simulink library "carnotUIBK"  (R2018b)
settings: Solver=VariableStepAuto  StartTime=0.0  StopTime=10.0  RelTol=1e-3  EnableMultiTasking=on
values from neighbouring files (symbols this model uses):
  A = 7*10*2    (= 140)    [theta_ground_v1.m]    (also in xlswrite1.m = num2cell(data))
  amb_factor = 1    [DOOR.m]    (also in WALL.m; WINDOW.m = 0)
  area = obj.width * obj.height    [DOOR.m]    (also in RES.m = []; ROOM.m = 0; THERMALZONE.m = area + room(kk).area; WALL.m = area - obj.doors(jj).calc_area())
  B = A/(0.5 * P)    (= 8.23529411765)    [theta_ground_v1.m]
  boundary = BOUNDARY()    [BUILDING.m]    (also in WALL.m = '')
  building = obj    [BUILDING.m]    (also in create_building_automatic.m = building.save(); ini_building_automatic.m = building.add_variant_hvac(building.variant_hvac, hvac); load_building_automatic.m = building.save())
  C = zeros(1,length(d)+1)    [CONSTRUCTION.m]    (also in DOOR.m = [0 0 0]; WALL.m = [0 0 0]; WINDOW.m = [0 0 0])
  control = 2    [GAIN.m]    (also in GAINS.m)
  cp = str2num(value)    [CONSTRUCTION.m]
  height = 0    [DOOR.m]    (also in ROOM.m; THERMALZONE.m; WALL.m; WINDOW.m)
  p = [timevec_weather weather(:,12)]    [BOUNDARY.m]    (also in WEATHER.m = 0; init_carnotUIBK.m = cell2mat(carnotUIBKpaths(i,2)))
  rho = str2num(value)    [CONSTRUCTION.m]    (also in theta_ground_v1.m = 2000)
  type = 1    [CONSTRUCTION.m]    (also in GAINS.m = raw_moisture{ii,3}; STRUCTURE.m = 0)
  view_factor = 1    [DOOR.m]    (also in WINDOW.m = 0)
  wall = []    [ROOM.m]
  z = obj.Z    [WALL.m]    (also in theta_ground_v1.m = 0)
  zone = obj.zone(ind)    [THERMALZONE.m]
undefined symbols (not defined in the file or in its folder): const, Dd, get_building, pos, Qdot_C, Qdot_H, Qdot_I_electricity, Qdot_I_light, Qdot_I_person, Qdot_S, Qdot_T_ground, Qdot_T_neighbour, Qdot_T_opaque, Qdot_T_window, Qdot_V_infiltration, Qdot_V_mech, Qdot_V_window, r_frame, solar_ratio, solar_ratio1, solar_ratio2, Tc, Tr, Ts, Uvalue, wallsurface, window, window_height, window_heigth, window_width, windowsurface, x_CO2, x_H2O, x_VOC
libraries: carnot x104, simulink x16, $bdroot x16, simulink_extras x14
(part 5 of 12)

== system carnotUIBK/HVAC/HVAC_1001_electrical heaters/electrical heater zone 6 ==
  temperature setpoint : Inport
  temperature room : Inport  Port=2
  Enable : EnablePort
  " " : Constant  Value=0
  "   " : Constant  Value=zeros(1,15)
  Bus Creator1 : BusCreator  Inputs=2
  Bus Selector5 : BusSelector  OutputSignals=Ts
  Integrator : Integrator
  Mux1 : Mux  Inputs=[1 1 15 1 1]
  PID : simulink/Continuous/PID Controller  Controller=PI  Form=Ideal  TimeDomain=Continuous-time  SampleTime=-1  IntegratorMethod=Forward Euler  FilterMethod=Forward Euler  ControllerParametersSource=internal  P=Kp  I=1/(Tn*60)  D=0  UseFilter=on  N=100  TunerSelectOption=Transfer Function Based (PID Tuner App)  InitialConditionSource=internal  InitialConditionForIntegrator=0  InitialConditionForFilter=0  DifferentiatorICPrevScaledInput=0  ExternalReset=none  TrackingMode=off  Kt=1  LimitOutput=on  UpperSaturationLimit=1  LowerSaturationLimit=0  LinearizeAsGain=off  AntiWindupMode=clamping  Kb=1  POutMin=[]  POutMax=[]  IOutMin=[]  IOutMax=[]  DOutMin=[]  DOutMax=[]  NOutMin=[]  NOutMax=[]  SumOutMin=[]  SumOutMax=[]  SaturationOutMin=[]  SaturationOutMax=[]  PParamMin=[]  PParamMax=[]  IParamMin=[]  IParamMax=[]  DParamMin=[]  DParamMax=[]  NParamMin=[]  NParamMax=[]  KbParamMin=[]  KbParamMax=[]  KtParamMin=[]  KtParamMax=[]  KbOutMin=[]  KbOutMax=[]  KtOutMin=[]  KtOutMax=[]  IntegratorOutMin=[]  IntegratorOutMax=[]  FilterOutMin=[]  FilterOutMax=[]  SumI1OutMin=[]  SumI1OutMax=[]  SumI2OutMin=[]  SumI2OutMax=[]  SumI3OutMin=[]  SumI3OutMax=[]  SumI4OutMin=[]  SumI4OutMax=[]  SumDOutMin=[]  SumDOutMax=[]  DifferentiatorOutMin=[]  DifferentiatorOutMax=[]  FilterDiffOutCoefMin=[]  FilterDiffOutCoefMax=[]  ReciprocalOutMin=[]  ReciprocalOutMax=[]  SumDenOutMin=[]  SumDenOutMax=[]  SumNumOutMin=[]  SumNumOutMax=[]  DivideOutMin=[]  DivideOutMax=[]  IntegratorContinuousStateAttributes=''  IntegratorStateMustResolveToSignalObject=off  IntegratorRTWStateStorageClass=Auto  FilterContinuousStateAttributes=''  FilterStateMustResolveToSignalObject=off  FilterRTWStateStorageClass=Auto  ParallelPVariant=Passthrough  IdealPVariant=InternalParameters  IVariant=InternalParameters  DVariant=Disabled  IntegratorVariant=Continuous  SatVariant=Enabled  AWVariant=ContClampingIdeal  PCopyVariant=InternalParamsIdeal  TRVariant=Disabled  FdbkBlocksVariant=Forward  IdealPFdbkVariant=Disabled  SatFdbkVariant=Disabled  DerivativeFilterVariant=Disabled  NVariant=Disabled  NCopyVariant=Disabled_SignalSpec  FilterICVariant=Disabled  IntegratorICVariant=InternalICs  ExternalResetVariant=Disabled  TRSumVariant=Passthrough  SumFdbkVariant=Disabled  SumVariant=Sum_PI
  Product : Product
  Sum13 : Sum  Inputs=|+-
  Transfer Fcn (with initial states) : Subsystem  mask(Transfer Function with Initial States){N=[1], D=[timeconst 1], X0=0}
      mask prompts: N "Numerator:"; D "Denominator:"; X0 "Initial conditions:"
      mask help: Vector expressions for numerator, and denominator. Coefficients are in descending powers of s.
      mask init:
      | [A,B,C,Dd]=tf2ss(N,D);if (isempty(X0));[m,n]=size(A);X0=zeros(1,m); end;
      mask Help: Specify the initial states for the transfer function.  The state ordering is determined by the m-file tf2ss.  There is no unique mapping of the states in a transfer function to states in a state-space representation.  However, tf2ss will consistently use the same mapping for a given transfer function.
      mask Display: dpoly(N,D,'s')
  convective : Gain  Gain=s_conv  SaturateOnIntegerOverflow=on  OutDataTypeStr=Inherit: Same as input  ParamDataTypeStr=Inherit: Same as input
  maximal power : Constant  Value=max_power
  radiative : Gain  Gain=1-s_conv  SaturateOnIntegerOverflow=on  OutDataTypeStr=Inherit: Same as input  ParamDataTypeStr=Inherit: Same as input
  "[S]" : Outport
  "[HVAC]" : Outport  Port=2
  wires:
  Bus Creator1/1 -> "[HVAC]"/1
  Integrator/1 -> Bus Creator1/2  "heating energy"
  temperature setpoint/1 -> Sum13/1
  Bus Selector5/1 -> Sum13/2  "<Ts>"
  Product/1 -> Mux1/4, Integrator/1, Bus Creator1/1, radiative/1, convective/1  "heating power"
  "   "/1 -> Mux1/3
  radiative/1 -> Mux1/2
  temperature room/1 -> Bus Selector5/1
  maximal power/1 -> Product/2
  PID/1 -> Transfer Fcn (with initial states)/1(In1)
  convective/1 -> Mux1/1
  Mux1/1 -> "[S]"/1
  " "/1 -> Mux1/5
  Transfer Fcn (with initial states)/1(Out1) -> Product/1
  Sum13/1 -> PID/1

== system carnotUIBK/HVAC/HVAC_1001_electrical heaters/electrical heater zone 7 ==
  temperature setpoint : Inport
  temperature room : Inport  Port=2
  Enable : EnablePort
  " " : Constant  Value=0
  "   " : Constant  Value=zeros(1,15)
  Bus Creator1 : BusCreator  Inputs=2
  Bus Selector5 : BusSelector  OutputSignals=Ts
  Integrator : Integrator
  Mux1 : Mux  Inputs=[1 1 15 1 1]
  PID : simulink/Continuous/PID Controller  Controller=PI  Form=Ideal  TimeDomain=Continuous-time  SampleTime=-1  IntegratorMethod=Forward Euler  FilterMethod=Forward Euler  ControllerParametersSource=internal  P=Kp  I=1/(Tn*60)  D=0  UseFilter=on  N=100  TunerSelectOption=Transfer Function Based (PID Tuner App)  InitialConditionSource=internal  InitialConditionForIntegrator=0  InitialConditionForFilter=0  DifferentiatorICPrevScaledInput=0  ExternalReset=none  TrackingMode=off  Kt=1  LimitOutput=on  UpperSaturationLimit=1  LowerSaturationLimit=0  LinearizeAsGain=off  AntiWindupMode=clamping  Kb=1  POutMin=[]  POutMax=[]  IOutMin=[]  IOutMax=[]  DOutMin=[]  DOutMax=[]  NOutMin=[]  NOutMax=[]  SumOutMin=[]  SumOutMax=[]  SaturationOutMin=[]  SaturationOutMax=[]  PParamMin=[]  PParamMax=[]  IParamMin=[]  IParamMax=[]  DParamMin=[]  DParamMax=[]  NParamMin=[]  NParamMax=[]  KbParamMin=[]  KbParamMax=[]  KtParamMin=[]  KtParamMax=[]  KbOutMin=[]  KbOutMax=[]  KtOutMin=[]  KtOutMax=[]  IntegratorOutMin=[]  IntegratorOutMax=[]  FilterOutMin=[]  FilterOutMax=[]  SumI1OutMin=[]  SumI1OutMax=[]  SumI2OutMin=[]  SumI2OutMax=[]  SumI3OutMin=[]  SumI3OutMax=[]  SumI4OutMin=[]  SumI4OutMax=[]  SumDOutMin=[]  SumDOutMax=[]  DifferentiatorOutMin=[]  DifferentiatorOutMax=[]  FilterDiffOutCoefMin=[]  FilterDiffOutCoefMax=[]  ReciprocalOutMin=[]  ReciprocalOutMax=[]  SumDenOutMin=[]  SumDenOutMax=[]  SumNumOutMin=[]  SumNumOutMax=[]  DivideOutMin=[]  DivideOutMax=[]  IntegratorContinuousStateAttributes=''  IntegratorStateMustResolveToSignalObject=off  IntegratorRTWStateStorageClass=Auto  FilterContinuousStateAttributes=''  FilterStateMustResolveToSignalObject=off  FilterRTWStateStorageClass=Auto  ParallelPVariant=Passthrough  IdealPVariant=InternalParameters  IVariant=InternalParameters  DVariant=Disabled  IntegratorVariant=Continuous  SatVariant=Enabled  AWVariant=ContClampingIdeal  PCopyVariant=InternalParamsIdeal  TRVariant=Disabled  FdbkBlocksVariant=Forward  IdealPFdbkVariant=Disabled  SatFdbkVariant=Disabled  DerivativeFilterVariant=Disabled  NVariant=Disabled  NCopyVariant=Disabled_SignalSpec  FilterICVariant=Disabled  IntegratorICVariant=InternalICs  ExternalResetVariant=Disabled  TRSumVariant=Passthrough  SumFdbkVariant=Disabled  SumVariant=Sum_PI
  Product : Product
  Sum13 : Sum  Inputs=|+-
  Transfer Fcn (with initial states) : Subsystem  mask(Transfer Function with Initial States){N=[1], D=[timeconst 1], X0=0}
      mask prompts: N "Numerator:"; D "Denominator:"; X0 "Initial conditions:"
      mask help: Vector expressions for numerator, and denominator. Coefficients are in descending powers of s.
      mask init:
      | [A,B,C,Dd]=tf2ss(N,D);if (isempty(X0));[m,n]=size(A);X0=zeros(1,m); end;
      mask Help: Specify the initial states for the transfer function.  The state ordering is determined by the m-file tf2ss.  There is no unique mapping of the states in a transfer function to states in a state-space representation.  However, tf2ss will consistently use the same mapping for a given transfer function.
      mask Display: dpoly(N,D,'s')
  convective : Gain  Gain=s_conv  SaturateOnIntegerOverflow=on  OutDataTypeStr=Inherit: Same as input  ParamDataTypeStr=Inherit: Same as input
  maximal power : Constant  Value=max_power
  radiative : Gain  Gain=1-s_conv  SaturateOnIntegerOverflow=on  OutDataTypeStr=Inherit: Same as input  ParamDataTypeStr=Inherit: Same as input
  "[S]" : Outport
  "[HVAC]" : Outport  Port=2
  wires:
  Sum13/1 -> PID/1
  Transfer Fcn (with initial states)/1(Out1) -> Product/1
  " "/1 -> Mux1/5
  Mux1/1 -> "[S]"/1
  convective/1 -> Mux1/1
  PID/1 -> Transfer Fcn (with initial states)/1(In1)
  maximal power/1 -> Product/2
  temperature room/1 -> Bus Selector5/1
  radiative/1 -> Mux1/2
  "   "/1 -> Mux1/3
  Product/1 -> convective/1, radiative/1, Bus Creator1/1, Integrator/1, Mux1/4  "heating power"
  Bus Selector5/1 -> Sum13/2  "<Ts>"
  temperature setpoint/1 -> Sum13/1
  Integrator/1 -> Bus Creator1/2  "heating energy"
  Bus Creator1/1 -> "[HVAC]"/1

== system carnotUIBK/HVAC/HVAC_1001_electrical heaters/electrical heater zone 8 ==
  temperature setpoint : Inport
  temperature room : Inport  Port=2
  Enable : EnablePort
  " " : Constant  Value=0
  "   " : Constant  Value=zeros(1,15)
  Bus Creator1 : BusCreator  Inputs=2
  Bus Selector5 : BusSelector  OutputSignals=Ts
  Integrator : Integrator
  Mux1 : Mux  Inputs=[1 1 15 1 1]
  PID : simulink/Continuous/PID Controller  Controller=PI  Form=Ideal  TimeDomain=Continuous-time  SampleTime=-1  IntegratorMethod=Forward Euler  FilterMethod=Forward Euler  ControllerParametersSource=internal  P=Kp  I=1/(Tn*60)  D=0  UseFilter=on  N=100  TunerSelectOption=Transfer Function Based (PID Tuner App)  InitialConditionSource=internal  InitialConditionForIntegrator=0  InitialConditionForFilter=0  DifferentiatorICPrevScaledInput=0  ExternalReset=none  TrackingMode=off  Kt=1  LimitOutput=on  UpperSaturationLimit=1  LowerSaturationLimit=0  LinearizeAsGain=off  AntiWindupMode=clamping  Kb=1  POutMin=[]  POutMax=[]  IOutMin=[]  IOutMax=[]  DOutMin=[]  DOutMax=[]  NOutMin=[]  NOutMax=[]  SumOutMin=[]  SumOutMax=[]  SaturationOutMin=[]  SaturationOutMax=[]  PParamMin=[]  PParamMax=[]  IParamMin=[]  IParamMax=[]  DParamMin=[]  DParamMax=[]  NParamMin=[]  NParamMax=[]  KbParamMin=[]  KbParamMax=[]  KtParamMin=[]  KtParamMax=[]  KbOutMin=[]  KbOutMax=[]  KtOutMin=[]  KtOutMax=[]  IntegratorOutMin=[]  IntegratorOutMax=[]  FilterOutMin=[]  FilterOutMax=[]  SumI1OutMin=[]  SumI1OutMax=[]  SumI2OutMin=[]  SumI2OutMax=[]  SumI3OutMin=[]  SumI3OutMax=[]  SumI4OutMin=[]  SumI4OutMax=[]  SumDOutMin=[]  SumDOutMax=[]  DifferentiatorOutMin=[]  DifferentiatorOutMax=[]  FilterDiffOutCoefMin=[]  FilterDiffOutCoefMax=[]  ReciprocalOutMin=[]  ReciprocalOutMax=[]  SumDenOutMin=[]  SumDenOutMax=[]  SumNumOutMin=[]  SumNumOutMax=[]  DivideOutMin=[]  DivideOutMax=[]  IntegratorContinuousStateAttributes=''  IntegratorStateMustResolveToSignalObject=off  IntegratorRTWStateStorageClass=Auto  FilterContinuousStateAttributes=''  FilterStateMustResolveToSignalObject=off  FilterRTWStateStorageClass=Auto  ParallelPVariant=Passthrough  IdealPVariant=InternalParameters  IVariant=InternalParameters  DVariant=Disabled  IntegratorVariant=Continuous  SatVariant=Enabled  AWVariant=ContClampingIdeal  PCopyVariant=InternalParamsIdeal  TRVariant=Disabled  FdbkBlocksVariant=Forward  IdealPFdbkVariant=Disabled  SatFdbkVariant=Disabled  DerivativeFilterVariant=Disabled  NVariant=Disabled  NCopyVariant=Disabled_SignalSpec  FilterICVariant=Disabled  IntegratorICVariant=InternalICs  ExternalResetVariant=Disabled  TRSumVariant=Passthrough  SumFdbkVariant=Disabled  SumVariant=Sum_PI
  Product : Product
  Sum13 : Sum  Inputs=|+-
  Transfer Fcn (with initial states) : Subsystem  mask(Transfer Function with Initial States){N=[1], D=[timeconst 1], X0=0}
      mask prompts: N "Numerator:"; D "Denominator:"; X0 "Initial conditions:"
      mask help: Vector expressions for numerator, and denominator. Coefficients are in descending powers of s.
      mask init:
      | [A,B,C,Dd]=tf2ss(N,D);if (isempty(X0));[m,n]=size(A);X0=zeros(1,m); end;
      mask Help: Specify the initial states for the transfer function.  The state ordering is determined by the m-file tf2ss.  There is no unique mapping of the states in a transfer function to states in a state-space representation.  However, tf2ss will consistently use the same mapping for a given transfer function.
      mask Display: dpoly(N,D,'s')
  convective : Gain  Gain=s_conv  SaturateOnIntegerOverflow=on  OutDataTypeStr=Inherit: Same as input  ParamDataTypeStr=Inherit: Same as input
  maximal power : Constant  Value=max_power
  radiative : Gain  Gain=1-s_conv  SaturateOnIntegerOverflow=on  OutDataTypeStr=Inherit: Same as input  ParamDataTypeStr=Inherit: Same as input
  "[S]" : Outport
  "[HVAC]" : Outport  Port=2
  wires:
  Bus Creator1/1 -> "[HVAC]"/1
  Integrator/1 -> Bus Creator1/2  "heating energy"
  temperature setpoint/1 -> Sum13/1
  Bus Selector5/1 -> Sum13/2  "<Ts>"
  Product/1 -> Mux1/4, Integrator/1, Bus Creator1/1, radiative/1, convective/1  "heating power"
  "   "/1 -> Mux1/3
  radiative/1 -> Mux1/2
  temperature room/1 -> Bus Selector5/1
  maximal power/1 -> Product/2
  PID/1 -> Transfer Fcn (with initial states)/1(In1)
  convective/1 -> Mux1/1
  Mux1/1 -> "[S]"/1
  " "/1 -> Mux1/5
  Transfer Fcn (with initial states)/1(Out1) -> Product/1
  Sum13/1 -> PID/1

== system carnotUIBK/HVAC/HVAC_1001_electrical heaters/electrical heater zone 9 ==
  temperature setpoint : Inport
  temperature room : Inport  Port=2
  Enable : EnablePort
  " " : Constant  Value=0
  "   " : Constant  Value=zeros(1,15)
  Bus Creator1 : BusCreator  Inputs=2
  Bus Selector5 : BusSelector  OutputSignals=Ts
  Integrator : Integrator
  Mux1 : Mux  Inputs=[1 1 15 1 1]
  PID : simulink/Continuous/PID Controller  Controller=PI  Form=Ideal  TimeDomain=Continuous-time  SampleTime=-1  IntegratorMethod=Forward Euler  FilterMethod=Forward Euler  ControllerParametersSource=internal  P=Kp  I=1/(Tn*60)  D=0  UseFilter=on  N=100  TunerSelectOption=Transfer Function Based (PID Tuner App)  InitialConditionSource=internal  InitialConditionForIntegrator=0  InitialConditionForFilter=0  DifferentiatorICPrevScaledInput=0  ExternalReset=none  TrackingMode=off  Kt=1  LimitOutput=on  UpperSaturationLimit=1  LowerSaturationLimit=0  LinearizeAsGain=off  AntiWindupMode=clamping  Kb=1  POutMin=[]  POutMax=[]  IOutMin=[]  IOutMax=[]  DOutMin=[]  DOutMax=[]  NOutMin=[]  NOutMax=[]  SumOutMin=[]  SumOutMax=[]  SaturationOutMin=[]  SaturationOutMax=[]  PParamMin=[]  PParamMax=[]  IParamMin=[]  IParamMax=[]  DParamMin=[]  DParamMax=[]  NParamMin=[]  NParamMax=[]  KbParamMin=[]  KbParamMax=[]  KtParamMin=[]  KtParamMax=[]  KbOutMin=[]  KbOutMax=[]  KtOutMin=[]  KtOutMax=[]  IntegratorOutMin=[]  IntegratorOutMax=[]  FilterOutMin=[]  FilterOutMax=[]  SumI1OutMin=[]  SumI1OutMax=[]  SumI2OutMin=[]  SumI2OutMax=[]  SumI3OutMin=[]  SumI3OutMax=[]  SumI4OutMin=[]  SumI4OutMax=[]  SumDOutMin=[]  SumDOutMax=[]  DifferentiatorOutMin=[]  DifferentiatorOutMax=[]  FilterDiffOutCoefMin=[]  FilterDiffOutCoefMax=[]  ReciprocalOutMin=[]  ReciprocalOutMax=[]  SumDenOutMin=[]  SumDenOutMax=[]  SumNumOutMin=[]  SumNumOutMax=[]  DivideOutMin=[]  DivideOutMax=[]  IntegratorContinuousStateAttributes=''  IntegratorStateMustResolveToSignalObject=off  IntegratorRTWStateStorageClass=Auto  FilterContinuousStateAttributes=''  FilterStateMustResolveToSignalObject=off  FilterRTWStateStorageClass=Auto  ParallelPVariant=Passthrough  IdealPVariant=InternalParameters  IVariant=InternalParameters  DVariant=Disabled  IntegratorVariant=Continuous  SatVariant=Enabled  AWVariant=ContClampingIdeal  PCopyVariant=InternalParamsIdeal  TRVariant=Disabled  FdbkBlocksVariant=Forward  IdealPFdbkVariant=Disabled  SatFdbkVariant=Disabled  DerivativeFilterVariant=Disabled  NVariant=Disabled  NCopyVariant=Disabled_SignalSpec  FilterICVariant=Disabled  IntegratorICVariant=InternalICs  ExternalResetVariant=Disabled  TRSumVariant=Passthrough  SumFdbkVariant=Disabled  SumVariant=Sum_PI
  Product : Product
  Sum13 : Sum  Inputs=|+-
  Transfer Fcn (with initial states) : Subsystem  mask(Transfer Function with Initial States){N=[1], D=[timeconst 1], X0=0}
      mask prompts: N "Numerator:"; D "Denominator:"; X0 "Initial conditions:"
      mask help: Vector expressions for numerator, and denominator. Coefficients are in descending powers of s.
      mask init:
      | [A,B,C,Dd]=tf2ss(N,D);if (isempty(X0));[m,n]=size(A);X0=zeros(1,m); end;
      mask Help: Specify the initial states for the transfer function.  The state ordering is determined by the m-file tf2ss.  There is no unique mapping of the states in a transfer function to states in a state-space representation.  However, tf2ss will consistently use the same mapping for a given transfer function.
      mask Display: dpoly(N,D,'s')
  convective : Gain  Gain=s_conv  SaturateOnIntegerOverflow=on  OutDataTypeStr=Inherit: Same as input  ParamDataTypeStr=Inherit: Same as input
  maximal power : Constant  Value=max_power
  radiative : Gain  Gain=1-s_conv  SaturateOnIntegerOverflow=on  OutDataTypeStr=Inherit: Same as input  ParamDataTypeStr=Inherit: Same as input
  "[S]" : Outport
  "[HVAC]" : Outport  Port=2
  wires:
  Sum13/1 -> PID/1
  Transfer Fcn (with initial states)/1(Out1) -> Product/1
  " "/1 -> Mux1/5
  Mux1/1 -> "[S]"/1
  convective/1 -> Mux1/1
  PID/1 -> Transfer Fcn (with initial states)/1(In1)
  maximal power/1 -> Product/2
  temperature room/1 -> Bus Selector5/1
  radiative/1 -> Mux1/2
  "   "/1 -> Mux1/3
  Product/1 -> convective/1, radiative/1, Bus Creator1/1, Integrator/1, Mux1/4  "heating power"
  Bus Selector5/1 -> Sum13/2  "<Ts>"
  temperature setpoint/1 -> Sum13/1
  Integrator/1 -> Bus Creator1/2  "heating energy"
  Bus Creator1/1 -> "[HVAC]"/1

== system carnotUIBK/HVAC/HVAC_1_PHPP/Transfer Fcn (with initial states) ==
  In1 : Inport
  State Space : StateSpace  A=A  B=B  C=C  D=Dd  InitialCondition=X0
  Out1 : Outport  InitialOutput=0
  wires:
  State Space/1 -> Out1/1
  In1/1 -> State Space/1

== system carnotUIBK/HVAC/HVAC_1_PHPP/Transfer Fcn (with initial states)1 ==
  In1 : Inport
  State Space : StateSpace  A=A  B=B  C=C  D=Dd  InitialCondition=X0
  Out1 : Outport  InitialOutput=0
  wires:
  State Space/1 -> Out1/1
  In1/1 -> State Space/1

== system carnotUIBK/HVAC/HVAC_2001_ventilation system simple/ventilation_zone 1 ==
  note: ASSUMPTION: mdot_air_in = mdot_air_out !
  note: AIR VENTILATION outdoors - indoors
  note: x_sup = x_amb + (x_ext - x_amb) * eta_x
  AIB : Inport
  WDB : Inport  Port=2
  Vdot : Inport  Port=3
  Enable : EnablePort
  "\"air\"" : Constant  Value=2
  "1/h -> 1/s" : Gain  Gain=1/3600  SaturateOnIntegerOverflow=on  OutDataTypeStr=Inherit: Same as input  ParamDataTypeStr=Inherit: Same as input
  Bus Creator1 : BusCreator  Inputs=2
  Bus Selector : BusSelector  OutputSignals=Temperature_Ambient,Relative_Humidity,Station_Pressure
  Bus Selector1 : BusSelector  OutputSignals=Tc,x_H2O,x_CO2
  Constant : Constant  Value=zeros(1,2)
  Constant1 : Constant  Value=zeros(1,5)
  Constant2 : Constant  Value=zeros(1,7)
  Constant3 : Constant  Value=1-eta
  Constant4 : Constant  Value=0
  Constant5 : Constant  Value=eta_x
  Density : carnot/Basic/Material_Properties/Density  VariantControl=CarlibClassic  INPUTARGUMENTS=state variables (classic)  DEBUGLEVEL=NOLEVEL  MAXTOTALWARNINGS=inf  MAXCONSECUTIVEWARNINGS=inf  WRITETOFILE=0  FILENAME='errors.txt'
  Fcn : Fcn  Expr=u / (1+u)
  Fcn1 : Fcn  Expr=u / (1+u)
  Integrator : Integrator
  Mux1 : Mux  Inputs=[1 1]
  Mux3 : Mux  Inputs=[1 2 1 1 1 5 1 7]
  Mux4 : Mux  Inputs=2
  Product1 : Product  SaturateOnIntegerOverflow=on  InputSameDT=on  OutDataTypeStr=Inherit: Same as first input
  Product2 : Product  SaturateOnIntegerOverflow=on  InputSameDT=on  OutDataTypeStr=Inherit: Same as first input
  Product3 : Product  SaturateOnIntegerOverflow=on  InputSameDT=on  OutDataTypeStr=Inherit: Same as first input
  Product4 : Product  Inputs=4  SaturateOnIntegerOverflow=on  InputSameDT=on  OutDataTypeStr=Inherit: Same as first input
  RelHum2x : carnot/Basic/Material_Properties/RelHum2x
  Subsystem : Subsystem
  Sum : Sum  Inputs=-+  SaturateOnIntegerOverflow=on  InputSameDT=on  OutDataTypeStr=Inherit: Same as first input
  Sum1 : Sum  Inputs=-+  SaturateOnIntegerOverflow=on  InputSameDT=on  OutDataTypeStr=Inherit: Same as first input
  Sum2 : Sum  Inputs=++-  SaturateOnIntegerOverflow=on  InputSameDT=on  OutDataTypeStr=Inherit: Same as first input
  Terminator : Terminator
  cp Constant : Constant  Value=1006.8
  rho(CO2) / rho(air) * CO2norm (kg/kg) : Constant  Value=1.529*CO2norm
  "[S]" : Outport
  "[HVAC]" : Outport  Port=2
  wires:
  Fcn1/1 -> Sum2/1, Sum1/1
  Fcn/1 -> Sum1/2, Sum2/3
  Product2/1 -> Mux3/4  "mdot_H2O"
  Sum2/1 -> Product2/2  "x_sup"
  Product1/1 -> Sum2/2
  Sum1/1 -> Product1/2
  Constant5/1 -> Product1/1
  Subsystem/1(mdot_H2O) -> Terminator/1  "mdot_H2O"
  Constant4/1 -> Mux3/3
  Vdot/1 -> "1/h -> 1/s"/1
  Mux3/1 -> "[S]"/1
  Subsystem/2(mdot_CO2) -> Mux3/5  "mdot_CO2"
  WDB/1 -> Bus Selector/1
  AIB/1 -> Bus Selector1/1
  Density/1 -> Product3/2
  Bus Selector/3 -> RelHum2x/2, Density/2  "<Station_Pressure>"
  Bus Selector/2 -> RelHum2x/3  "<Relative_Humidity>"
  Bus Selector/1 -> RelHum2x/1, Density/1, Sum/2  "<Temperature_Ambient>"
  RelHum2x/1 -> Density/4, Mux4/1, Fcn1/1  "x_H2O"
  "\"air\""/1 -> Density/3
  Mux1/1 -> Subsystem/2(x_in)  "[x_H2O, x_CO2]_in"
  Bus Selector1/1 -> Sum/1  "<Tc>"
  Mux4/1 -> Subsystem/3(x_out)
  rho(CO2) / rho(air) * CO2norm (kg/kg)/1 -> Mux4/2  "x_CO2"
  Sum/1 -> Product4/2  "dT"
  cp Constant/1 -> Product4/3  "cp"
  Product3/1 -> Product4/4, Product2/1, Subsystem/1(mdot_air)
  Bus Selector1/2 -> Mux1/1, Fcn/1  "<x_H2O>"
  Bus Selector1/3 -> Mux1/2  "<x_CO2>"
  Constant/1 -> Mux3/2
  Constant1/1 -> Mux3/6
  Constant2/1 -> Mux3/8
  Constant3/1 -> Product4/1
  "1/h -> 1/s"/1 -> Product3/1
  Bus Creator1/1 -> "[HVAC]"/1
  Product4/1 -> Mux3/7, Integrator/1, Bus Creator1/1, Mux3/1  "ventilation power"
  Integrator/1 -> Bus Creator1/2  "ventilation energy"

== system carnotUIBK/HVAC/HVAC_2001_ventilation system simple/ventilation_zone 10 ==
  note: ASSUMPTION: mdot_air_in = mdot_air_out !
  note: AIR VENTILATION outdoors - indoors
  note: x_sup = x_amb + (x_ext - x_amb) * eta_x
  AIB : Inport
  WDB : Inport  Port=2
  Vdot : Inport  Port=3
  Enable : EnablePort
  "\"air\"" : Constant  Value=2
  "1/h -> 1/s" : Gain  Gain=1/3600  SaturateOnIntegerOverflow=on  OutDataTypeStr=Inherit: Same as input  ParamDataTypeStr=Inherit: Same as input
  Bus Creator1 : BusCreator  Inputs=2
  Bus Selector : BusSelector  OutputSignals=Temperature_Ambient,Relative_Humidity,Station_Pressure
  Bus Selector1 : BusSelector  OutputSignals=Tc,x_H2O,x_CO2
  Constant : Constant  Value=zeros(1,2)
  Constant1 : Constant  Value=zeros(1,5)
  Constant2 : Constant  Value=zeros(1,7)
  Constant3 : Constant  Value=1-eta
  Constant4 : Constant  Value=0
  Constant5 : Constant  Value=eta_x
  Density : carnot/Basic/Material_Properties/Density  VariantControl=CarlibClassic  INPUTARGUMENTS=state variables (classic)  DEBUGLEVEL=NOLEVEL  MAXTOTALWARNINGS=inf  MAXCONSECUTIVEWARNINGS=inf  WRITETOFILE=0  FILENAME='errors.txt'
  Fcn : Fcn  Expr=u / (1+u)
  Fcn1 : Fcn  Expr=u / (1+u)
  Integrator : Integrator
  Mux1 : Mux  Inputs=[1 1]
  Mux3 : Mux  Inputs=[1 2 1 1 1 5 1 7]
  Mux4 : Mux  Inputs=2
  Product1 : Product  SaturateOnIntegerOverflow=on  InputSameDT=on  OutDataTypeStr=Inherit: Same as first input
  Product2 : Product  SaturateOnIntegerOverflow=on  InputSameDT=on  OutDataTypeStr=Inherit: Same as first input
  Product3 : Product  SaturateOnIntegerOverflow=on  InputSameDT=on  OutDataTypeStr=Inherit: Same as first input
  Product4 : Product  Inputs=4  SaturateOnIntegerOverflow=on  InputSameDT=on  OutDataTypeStr=Inherit: Same as first input
  RelHum2x : carnot/Basic/Material_Properties/RelHum2x
  Subsystem : Subsystem
  Sum : Sum  Inputs=-+  SaturateOnIntegerOverflow=on  InputSameDT=on  OutDataTypeStr=Inherit: Same as first input
  Sum1 : Sum  Inputs=-+  SaturateOnIntegerOverflow=on  InputSameDT=on  OutDataTypeStr=Inherit: Same as first input
  Sum2 : Sum  Inputs=++-  SaturateOnIntegerOverflow=on  InputSameDT=on  OutDataTypeStr=Inherit: Same as first input
  Terminator : Terminator
  cp Constant : Constant  Value=1006.8
  rho(CO2) / rho(air) * CO2norm (kg/kg) : Constant  Value=1.529*CO2norm
  "[S]" : Outport
  "[HVAC]" : Outport  Port=2
  wires:
  Fcn1/1 -> Sum2/1, Sum1/1
  Fcn/1 -> Sum1/2, Sum2/3
  Product2/1 -> Mux3/4  "mdot_H2O"
  Sum2/1 -> Product2/2  "x_sup"
  Product1/1 -> Sum2/2
  Sum1/1 -> Product1/2
  Constant5/1 -> Product1/1
  Subsystem/1(mdot_H2O) -> Terminator/1  "mdot_H2O"
  Constant4/1 -> Mux3/3
  Vdot/1 -> "1/h -> 1/s"/1
  Mux3/1 -> "[S]"/1
  Subsystem/2(mdot_CO2) -> Mux3/5  "mdot_CO2"
  WDB/1 -> Bus Selector/1
  AIB/1 -> Bus Selector1/1
  Density/1 -> Product3/2
  Bus Selector/3 -> RelHum2x/2, Density/2  "<Station_Pressure>"
  Bus Selector/2 -> RelHum2x/3  "<Relative_Humidity>"
  Bus Selector/1 -> RelHum2x/1, Density/1, Sum/2  "<Temperature_Ambient>"
  RelHum2x/1 -> Density/4, Mux4/1, Fcn1/1  "x_H2O"
  "\"air\""/1 -> Density/3
  Mux1/1 -> Subsystem/2(x_in)  "[x_H2O, x_CO2]_in"
  Bus Selector1/1 -> Sum/1  "<Tc>"
  Mux4/1 -> Subsystem/3(x_out)
  rho(CO2) / rho(air) * CO2norm (kg/kg)/1 -> Mux4/2  "x_CO2"
  Sum/1 -> Product4/2  "dT"
  cp Constant/1 -> Product4/3  "cp"
  Product3/1 -> Product4/4, Product2/1, Subsystem/1(mdot_air)
  Bus Selector1/2 -> Mux1/1, Fcn/1  "<x_H2O>"
  Bus Selector1/3 -> Mux1/2  "<x_CO2>"
  Constant/1 -> Mux3/2
  Constant1/1 -> Mux3/6
  Constant2/1 -> Mux3/8
  Constant3/1 -> Product4/1
  "1/h -> 1/s"/1 -> Product3/1
  Bus Creator1/1 -> "[HVAC]"/1
  Product4/1 -> Mux3/7, Integrator/1, Bus Creator1/1, Mux3/1  "ventilation power"
  Integrator/1 -> Bus Creator1/2  "ventilation energy"

== system carnotUIBK/HVAC/HVAC_2001_ventilation system simple/ventilation_zone 2 ==
  note: x_sup = x_amb + (x_ext - x_amb) * eta_x
  note: AIR VENTILATION outdoors - indoors
  note: ASSUMPTION: mdot_air_in = mdot_air_out !
  AIB : Inport
  WDB : Inport  Port=2
  Vdot : Inport  Port=3
  Enable : EnablePort
  "\"air\"" : Constant  Value=2
  "1/h -> 1/s" : Gain  Gain=1/3600  SaturateOnIntegerOverflow=on  OutDataTypeStr=Inherit: Same as input  ParamDataTypeStr=Inherit: Same as input
  Bus Creator1 : BusCreator  Inputs=2
  Bus Selector : BusSelector  OutputSignals=Temperature_Ambient,Relative_Humidity,Station_Pressure
  Bus Selector1 : BusSelector  OutputSignals=Tc,x_H2O,x_CO2
  Constant : Constant  Value=zeros(1,2)
  Constant1 : Constant  Value=zeros(1,5)
  Constant2 : Constant  Value=zeros(1,7)
  Constant3 : Constant  Value=1-eta
  Constant4 : Constant  Value=0
  Constant5 : Constant  Value=eta_x
  Density : carnot/Basic/Material_Properties/Density  VariantControl=CarlibClassic  INPUTARGUMENTS=state variables (classic)  DEBUGLEVEL=NOLEVEL  MAXTOTALWARNINGS=inf  MAXCONSECUTIVEWARNINGS=inf  WRITETOFILE=0  FILENAME='errors.txt'
  Fcn : Fcn  Expr=u / (1+u)
  Fcn1 : Fcn  Expr=u / (1+u)
  Integrator : Integrator
  Mux1 : Mux  Inputs=[1 1]
  Mux3 : Mux  Inputs=[1 2 1 1 1 5 1 7]
  Mux4 : Mux  Inputs=2
  Product1 : Product  SaturateOnIntegerOverflow=on  InputSameDT=on  OutDataTypeStr=Inherit: Same as first input
  Product2 : Product  SaturateOnIntegerOverflow=on  InputSameDT=on  OutDataTypeStr=Inherit: Same as first input
  Product3 : Product  SaturateOnIntegerOverflow=on  InputSameDT=on  OutDataTypeStr=Inherit: Same as first input
  Product4 : Product  Inputs=4  SaturateOnIntegerOverflow=on  InputSameDT=on  OutDataTypeStr=Inherit: Same as first input
  RelHum2x : carnot/Basic/Material_Properties/RelHum2x
  Subsystem : Subsystem
  Sum : Sum  Inputs=-+  SaturateOnIntegerOverflow=on  InputSameDT=on  OutDataTypeStr=Inherit: Same as first input
  Sum1 : Sum  Inputs=-+  SaturateOnIntegerOverflow=on  InputSameDT=on  OutDataTypeStr=Inherit: Same as first input
  Sum2 : Sum  Inputs=++-  SaturateOnIntegerOverflow=on  InputSameDT=on  OutDataTypeStr=Inherit: Same as first input
  Terminator : Terminator
  cp Constant : Constant  Value=1006.8
  rho(CO2) / rho(air) * CO2norm (kg/kg) : Constant  Value=1.529*CO2norm
  "[S]" : Outport
  "[HVAC]" : Outport  Port=2
  wires:
  Integrator/1 -> Bus Creator1/2  "ventilation energy"
  Product4/1 -> Mux3/1, Bus Creator1/1, Integrator/1, Mux3/7  "ventilation power"
  Bus Creator1/1 -> "[HVAC]"/1
  "1/h -> 1/s"/1 -> Product3/1
  Constant3/1 -> Product4/1
  Constant2/1 -> Mux3/8
  Constant1/1 -> Mux3/6
  Constant/1 -> Mux3/2
  Bus Selector1/3 -> Mux1/2  "<x_CO2>"
  Bus Selector1/2 -> Fcn/1, Mux1/1  "<x_H2O>"
  Product3/1 -> Subsystem/1(mdot_air), Product2/1, Product4/4
  cp Constant/1 -> Product4/3  "cp"
  Sum/1 -> Product4/2  "dT"
  rho(CO2) / rho(air) * CO2norm (kg/kg)/1 -> Mux4/2  "x_CO2"
  Mux4/1 -> Subsystem/3(x_out)
  Bus Selector1/1 -> Sum/1  "<Tc>"
  Mux1/1 -> Subsystem/2(x_in)  "[x_H2O, x_CO2]_in"
  "\"air\""/1 -> Density/3
  RelHum2x/1 -> Fcn1/1, Mux4/1, Density/4  "x_H2O"
  Bus Selector/1 -> Sum/2, Density/1, RelHum2x/1  "<Temperature_Ambient>"
  Bus Selector/2 -> RelHum2x/3  "<Relative_Humidity>"
  Bus Selector/3 -> Density/2, RelHum2x/2  "<Station_Pressure>"
  Density/1 -> Product3/2
  AIB/1 -> Bus Selector1/1
  WDB/1 -> Bus Selector/1
  Subsystem/2(mdot_CO2) -> Mux3/5  "mdot_CO2"
  Mux3/1 -> "[S]"/1
  Vdot/1 -> "1/h -> 1/s"/1
  Constant4/1 -> Mux3/3
  Subsystem/1(mdot_H2O) -> Terminator/1  "mdot_H2O"
  Constant5/1 -> Product1/1
  Sum1/1 -> Product1/2
  Product1/1 -> Sum2/2
  Sum2/1 -> Product2/2  "x_sup"
  Product2/1 -> Mux3/4  "mdot_H2O"
  Fcn/1 -> Sum2/3, Sum1/2
  Fcn1/1 -> Sum1/1, Sum2/1

== system carnotUIBK/HVAC/HVAC_2001_ventilation system simple/ventilation_zone 3 ==
  note: ASSUMPTION: mdot_air_in = mdot_air_out !
  note: AIR VENTILATION outdoors - indoors
  note: x_sup = x_amb + (x_ext - x_amb) * eta_x
  AIB : Inport
  WDB : Inport  Port=2
  Vdot : Inport  Port=3
  Enable : EnablePort
  "\"air\"" : Constant  Value=2
  "1/h -> 1/s" : Gain  Gain=1/3600  SaturateOnIntegerOverflow=on  OutDataTypeStr=Inherit: Same as input  ParamDataTypeStr=Inherit: Same as input
  Bus Creator1 : BusCreator  Inputs=2
  Bus Selector : BusSelector  OutputSignals=Temperature_Ambient,Relative_Humidity,Station_Pressure
  Bus Selector1 : BusSelector  OutputSignals=Tc,x_H2O,x_CO2
  Constant : Constant  Value=zeros(1,2)
  Constant1 : Constant  Value=zeros(1,5)
  Constant2 : Constant  Value=zeros(1,7)
  Constant3 : Constant  Value=1-eta
  Constant4 : Constant  Value=0
  Constant5 : Constant  Value=eta_x
  Density : carnot/Basic/Material_Properties/Density  VariantControl=CarlibClassic  INPUTARGUMENTS=state variables (classic)  DEBUGLEVEL=NOLEVEL  MAXTOTALWARNINGS=inf  MAXCONSECUTIVEWARNINGS=inf  WRITETOFILE=0  FILENAME='errors.txt'
  Fcn : Fcn  Expr=u / (1+u)
  Fcn1 : Fcn  Expr=u / (1+u)
  Integrator : Integrator
  Mux1 : Mux  Inputs=[1 1]
  Mux3 : Mux  Inputs=[1 2 1 1 1 5 1 7]
  Mux4 : Mux  Inputs=2
  Product1 : Product  SaturateOnIntegerOverflow=on  InputSameDT=on  OutDataTypeStr=Inherit: Same as first input
  Product2 : Product  SaturateOnIntegerOverflow=on  InputSameDT=on  OutDataTypeStr=Inherit: Same as first input
  Product3 : Product  SaturateOnIntegerOverflow=on  InputSameDT=on  OutDataTypeStr=Inherit: Same as first input
  Product4 : Product  Inputs=4  SaturateOnIntegerOverflow=on  InputSameDT=on  OutDataTypeStr=Inherit: Same as first input
  RelHum2x : carnot/Basic/Material_Properties/RelHum2x
  Subsystem : Subsystem
  Sum : Sum  Inputs=-+  SaturateOnIntegerOverflow=on  InputSameDT=on  OutDataTypeStr=Inherit: Same as first input
  Sum1 : Sum  Inputs=-+  SaturateOnIntegerOverflow=on  InputSameDT=on  OutDataTypeStr=Inherit: Same as first input
  Sum2 : Sum  Inputs=++-  SaturateOnIntegerOverflow=on  InputSameDT=on  OutDataTypeStr=Inherit: Same as first input
  Terminator : Terminator
  cp Constant : Constant  Value=1006.8
  rho(CO2) / rho(air) * CO2norm (kg/kg) : Constant  Value=1.529*CO2norm
  "[S]" : Outport
  "[HVAC]" : Outport  Port=2
  wires:
  Fcn1/1 -> Sum2/1, Sum1/1
  Fcn/1 -> Sum1/2, Sum2/3
  Product2/1 -> Mux3/4  "mdot_H2O"
  Sum2/1 -> Product2/2  "x_sup"
  Product1/1 -> Sum2/2
  Sum1/1 -> Product1/2
  Constant5/1 -> Product1/1
  Subsystem/1(mdot_H2O) -> Terminator/1  "mdot_H2O"
  Constant4/1 -> Mux3/3
  Vdot/1 -> "1/h -> 1/s"/1
  Mux3/1 -> "[S]"/1
  Subsystem/2(mdot_CO2) -> Mux3/5  "mdot_CO2"
  WDB/1 -> Bus Selector/1
  AIB/1 -> Bus Selector1/1
  Density/1 -> Product3/2
  Bus Selector/3 -> RelHum2x/2, Density/2  "<Station_Pressure>"
  Bus Selector/2 -> RelHum2x/3  "<Relative_Humidity>"
  Bus Selector/1 -> RelHum2x/1, Density/1, Sum/2  "<Temperature_Ambient>"
  RelHum2x/1 -> Density/4, Mux4/1, Fcn1/1  "x_H2O"
  "\"air\""/1 -> Density/3
  Mux1/1 -> Subsystem/2(x_in)  "[x_H2O, x_CO2]_in"
  Bus Selector1/1 -> Sum/1  "<Tc>"
  Mux4/1 -> Subsystem/3(x_out)
  rho(CO2) / rho(air) * CO2norm (kg/kg)/1 -> Mux4/2  "x_CO2"
  Sum/1 -> Product4/2  "dT"
  cp Constant/1 -> Product4/3  "cp"
  Product3/1 -> Product4/4, Product2/1, Subsystem/1(mdot_air)
  Bus Selector1/2 -> Mux1/1, Fcn/1  "<x_H2O>"
  Bus Selector1/3 -> Mux1/2  "<x_CO2>"
  Constant/1 -> Mux3/2
  Constant1/1 -> Mux3/6
  Constant2/1 -> Mux3/8
  Constant3/1 -> Product4/1
  "1/h -> 1/s"/1 -> Product3/1
  Bus Creator1/1 -> "[HVAC]"/1
  Product4/1 -> Mux3/7, Integrator/1, Bus Creator1/1, Mux3/1  "ventilation power"
  Integrator/1 -> Bus Creator1/2  "ventilation energy"

== system carnotUIBK/HVAC/HVAC_2001_ventilation system simple/ventilation_zone 4 ==
  note: ASSUMPTION: mdot_air_in = mdot_air_out !
  note: AIR VENTILATION outdoors - indoors
  note: x_sup = x_amb + (x_ext - x_amb) * eta_x
  AIB : Inport
  WDB : Inport  Port=2
  Vdot : Inport  Port=3
  Enable : EnablePort
  "\"air\"" : Constant  Value=2
  "1/h -> 1/s" : Gain  Gain=1/3600  SaturateOnIntegerOverflow=on  OutDataTypeStr=Inherit: Same as input  ParamDataTypeStr=Inherit: Same as input
  Bus Creator1 : BusCreator  Inputs=2
  Bus Selector : BusSelector  OutputSignals=Temperature_Ambient,Relative_Humidity,Station_Pressure
  Bus Selector1 : BusSelector  OutputSignals=Tc,x_H2O,x_CO2
  Constant : Constant  Value=zeros(1,2)
  Constant1 : Constant  Value=zeros(1,5)
  Constant2 : Constant  Value=zeros(1,7)
  Constant3 : Constant  Value=1-eta
  Constant4 : Constant  Value=0
  Constant5 : Constant  Value=eta_x
  Density : carnot/Basic/Material_Properties/Density  VariantControl=CarlibClassic  INPUTARGUMENTS=state variables (classic)  DEBUGLEVEL=NOLEVEL  MAXTOTALWARNINGS=inf  MAXCONSECUTIVEWARNINGS=inf  WRITETOFILE=0  FILENAME='errors.txt'
  Fcn : Fcn  Expr=u / (1+u)
  Fcn1 : Fcn  Expr=u / (1+u)
  Integrator : Integrator
  Mux1 : Mux  Inputs=[1 1]
  Mux3 : Mux  Inputs=[1 2 1 1 1 5 1 7]
  Mux4 : Mux  Inputs=2
  Product1 : Product  SaturateOnIntegerOverflow=on  InputSameDT=on  OutDataTypeStr=Inherit: Same as first input
  Product2 : Product  SaturateOnIntegerOverflow=on  InputSameDT=on  OutDataTypeStr=Inherit: Same as first input
  Product3 : Product  SaturateOnIntegerOverflow=on  InputSameDT=on  OutDataTypeStr=Inherit: Same as first input
  Product4 : Product  Inputs=4  SaturateOnIntegerOverflow=on  InputSameDT=on  OutDataTypeStr=Inherit: Same as first input
  RelHum2x : carnot/Basic/Material_Properties/RelHum2x
  Subsystem : Subsystem
  Sum : Sum  Inputs=-+  SaturateOnIntegerOverflow=on  InputSameDT=on  OutDataTypeStr=Inherit: Same as first input
  Sum1 : Sum  Inputs=-+  SaturateOnIntegerOverflow=on  InputSameDT=on  OutDataTypeStr=Inherit: Same as first input
  Sum2 : Sum  Inputs=++-  SaturateOnIntegerOverflow=on  InputSameDT=on  OutDataTypeStr=Inherit: Same as first input
  Terminator : Terminator
  cp Constant : Constant  Value=1006.8
  rho(CO2) / rho(air) * CO2norm (kg/kg) : Constant  Value=1.529*CO2norm
  "[S]" : Outport
  "[HVAC]" : Outport  Port=2
  wires:
  Fcn1/1 -> Sum2/1, Sum1/1
  Fcn/1 -> Sum1/2, Sum2/3
  Product2/1 -> Mux3/4  "mdot_H2O"
  Sum2/1 -> Product2/2  "x_sup"
  Product1/1 -> Sum2/2
  Sum1/1 -> Product1/2
  Constant5/1 -> Product1/1
  Subsystem/1(mdot_H2O) -> Terminator/1  "mdot_H2O"
  Constant4/1 -> Mux3/3
  Vdot/1 -> "1/h -> 1/s"/1
  Mux3/1 -> "[S]"/1
  Subsystem/2(mdot_CO2) -> Mux3/5  "mdot_CO2"
  WDB/1 -> Bus Selector/1
  AIB/1 -> Bus Selector1/1
  Density/1 -> Product3/2
  Bus Selector/3 -> RelHum2x/2, Density/2  "<Station_Pressure>"
  Bus Selector/2 -> RelHum2x/3  "<Relative_Humidity>"
  Bus Selector/1 -> RelHum2x/1, Density/1, Sum/2  "<Temperature_Ambient>"
  RelHum2x/1 -> Density/4, Mux4/1, Fcn1/1  "x_H2O"
  "\"air\""/1 -> Density/3
  Mux1/1 -> Subsystem/2(x_in)  "[x_H2O, x_CO2]_in"
  Bus Selector1/1 -> Sum/1  "<Tc>"
  Mux4/1 -> Subsystem/3(x_out)
  rho(CO2) / rho(air) * CO2norm (kg/kg)/1 -> Mux4/2  "x_CO2"
  Sum/1 -> Product4/2  "dT"
  cp Constant/1 -> Product4/3  "cp"
  Product3/1 -> Product4/4, Product2/1, Subsystem/1(mdot_air)
  Bus Selector1/2 -> Mux1/1, Fcn/1  "<x_H2O>"
  Bus Selector1/3 -> Mux1/2  "<x_CO2>"
  Constant/1 -> Mux3/2
  Constant1/1 -> Mux3/6
  Constant2/1 -> Mux3/8
  Constant3/1 -> Product4/1
  "1/h -> 1/s"/1 -> Product3/1
  Bus Creator1/1 -> "[HVAC]"/1
  Product4/1 -> Mux3/7, Integrator/1, Bus Creator1/1, Mux3/1  "ventilation power"
  Integrator/1 -> Bus Creator1/2  "ventilation energy"

== system carnotUIBK/HVAC/HVAC_2001_ventilation system simple/ventilation_zone 5 ==
  note: ASSUMPTION: mdot_air_in = mdot_air_out !
  note: AIR VENTILATION outdoors - indoors
  note: x_sup = x_amb + (x_ext - x_amb) * eta_x
  AIB : Inport
  WDB : Inport  Port=2
  Vdot : Inport  Port=3
  Enable : EnablePort
  "\"air\"" : Constant  Value=2
  "1/h -> 1/s" : Gain  Gain=1/3600  SaturateOnIntegerOverflow=on  OutDataTypeStr=Inherit: Same as input  ParamDataTypeStr=Inherit: Same as input
  Bus Creator1 : BusCreator  Inputs=2
  Bus Selector : BusSelector  OutputSignals=Temperature_Ambient,Relative_Humidity,Station_Pressure
  Bus Selector1 : BusSelector  OutputSignals=Tc,x_H2O,x_CO2
  Constant : Constant  Value=zeros(1,2)
  Constant1 : Constant  Value=zeros(1,5)
  Constant2 : Constant  Value=zeros(1,7)
  Constant3 : Constant  Value=1-eta
  Constant4 : Constant  Value=0
  Constant5 : Constant  Value=eta_x
  Density : carnot/Basic/Material_Properties/Density  VariantControl=CarlibClassic  INPUTARGUMENTS=state variables (classic)  DEBUGLEVEL=NOLEVEL  MAXTOTALWARNINGS=inf  MAXCONSECUTIVEWARNINGS=inf  WRITETOFILE=0  FILENAME='errors.txt'
  Fcn : Fcn  Expr=u / (1+u)
  Fcn1 : Fcn  Expr=u / (1+u)
  Integrator : Integrator
  Mux1 : Mux  Inputs=[1 1]
  Mux3 : Mux  Inputs=[1 2 1 1 1 5 1 7]
  Mux4 : Mux  Inputs=2
  Product1 : Product  SaturateOnIntegerOverflow=on  InputSameDT=on  OutDataTypeStr=Inherit: Same as first input
  Product2 : Product  SaturateOnIntegerOverflow=on  InputSameDT=on  OutDataTypeStr=Inherit: Same as first input
  Product3 : Product  SaturateOnIntegerOverflow=on  InputSameDT=on  OutDataTypeStr=Inherit: Same as first input
  Product4 : Product  Inputs=4  SaturateOnIntegerOverflow=on  InputSameDT=on  OutDataTypeStr=Inherit: Same as first input
  RelHum2x : carnot/Basic/Material_Properties/RelHum2x
  Subsystem : Subsystem
  Sum : Sum  Inputs=-+  SaturateOnIntegerOverflow=on  InputSameDT=on  OutDataTypeStr=Inherit: Same as first input
  Sum1 : Sum  Inputs=-+  SaturateOnIntegerOverflow=on  InputSameDT=on  OutDataTypeStr=Inherit: Same as first input
  Sum2 : Sum  Inputs=++-  SaturateOnIntegerOverflow=on  InputSameDT=on  OutDataTypeStr=Inherit: Same as first input
  Terminator : Terminator
  cp Constant : Constant  Value=1006.8
  rho(CO2) / rho(air) * CO2norm (kg/kg) : Constant  Value=1.529*CO2norm
  "[S]" : Outport
  "[HVAC]" : Outport  Port=2
  wires:
  Fcn1/1 -> Sum2/1, Sum1/1
  Fcn/1 -> Sum1/2, Sum2/3
  Product2/1 -> Mux3/4  "mdot_H2O"
  Sum2/1 -> Product2/2  "x_sup"
  Product1/1 -> Sum2/2
  Sum1/1 -> Product1/2
  Constant5/1 -> Product1/1
  Subsystem/1(mdot_H2O) -> Terminator/1  "mdot_H2O"
  Constant4/1 -> Mux3/3
  Vdot/1 -> "1/h -> 1/s"/1
  Mux3/1 -> "[S]"/1
  Subsystem/2(mdot_CO2) -> Mux3/5  "mdot_CO2"
  WDB/1 -> Bus Selector/1
  AIB/1 -> Bus Selector1/1
  Density/1 -> Product3/2
  Bus Selector/3 -> RelHum2x/2, Density/2  "<Station_Pressure>"
  Bus Selector/2 -> RelHum2x/3  "<Relative_Humidity>"
  Bus Selector/1 -> RelHum2x/1, Density/1, Sum/2  "<Temperature_Ambient>"
  RelHum2x/1 -> Density/4, Mux4/1, Fcn1/1  "x_H2O"
  "\"air\""/1 -> Density/3
  Mux1/1 -> Subsystem/2(x_in)  "[x_H2O, x_CO2]_in"
  Bus Selector1/1 -> Sum/1  "<Tc>"
  Mux4/1 -> Subsystem/3(x_out)
  rho(CO2) / rho(air) * CO2norm (kg/kg)/1 -> Mux4/2  "x_CO2"
  Sum/1 -> Product4/2  "dT"
  cp Constant/1 -> Product4/3  "cp"
  Product3/1 -> Product4/4, Product2/1, Subsystem/1(mdot_air)
  Bus Selector1/2 -> Mux1/1, Fcn/1  "<x_H2O>"
  Bus Selector1/3 -> Mux1/2  "<x_CO2>"
  Constant/1 -> Mux3/2
  Constant1/1 -> Mux3/6
  Constant2/1 -> Mux3/8
  Constant3/1 -> Product4/1
  "1/h -> 1/s"/1 -> Product3/1
  Bus Creator1/1 -> "[HVAC]"/1
  Product4/1 -> Mux3/7, Integrator/1, Bus Creator1/1, Mux3/1  "ventilation power"
  Integrator/1 -> Bus Creator1/2  "ventilation energy"

== system carnotUIBK/HVAC/HVAC_2001_ventilation system simple/ventilation_zone 6 ==
  note: ASSUMPTION: mdot_air_in = mdot_air_out !
  note: AIR VENTILATION outdoors - indoors
  note: x_sup = x_amb + (x_ext - x_amb) * eta_x
  AIB : Inport
  WDB : Inport  Port=2
  Vdot : Inport  Port=3
  Enable : EnablePort
  "\"air\"" : Constant  Value=2
  "1/h -> 1/s" : Gain  Gain=1/3600  SaturateOnIntegerOverflow=on  OutDataTypeStr=Inherit: Same as input  ParamDataTypeStr=Inherit: Same as input
  Bus Creator1 : BusCreator  Inputs=2
  Bus Selector : BusSelector  OutputSignals=Temperature_Ambient,Relative_Humidity,Station_Pressure
  Bus Selector1 : BusSelector  OutputSignals=Tc,x_H2O,x_CO2
  Constant : Constant  Value=zeros(1,2)
  Constant1 : Constant  Value=zeros(1,5)
  Constant2 : Constant  Value=zeros(1,7)
  Constant3 : Constant  Value=1-eta
  Constant4 : Constant  Value=0
  Constant5 : Constant  Value=eta_x
  Density : carnot/Basic/Material_Properties/Density  VariantControl=CarlibClassic  INPUTARGUMENTS=state variables (classic)  DEBUGLEVEL=NOLEVEL  MAXTOTALWARNINGS=inf  MAXCONSECUTIVEWARNINGS=inf  WRITETOFILE=0  FILENAME='errors.txt'
  Fcn : Fcn  Expr=u / (1+u)
  Fcn1 : Fcn  Expr=u / (1+u)
  Integrator : Integrator
  Mux1 : Mux  Inputs=[1 1]
  Mux3 : Mux  Inputs=[1 2 1 1 1 5 1 7]
  Mux4 : Mux  Inputs=2
  Product1 : Product  SaturateOnIntegerOverflow=on  InputSameDT=on  OutDataTypeStr=Inherit: Same as first input
  Product2 : Product  SaturateOnIntegerOverflow=on  InputSameDT=on  OutDataTypeStr=Inherit: Same as first input
  Product3 : Product  SaturateOnIntegerOverflow=on  InputSameDT=on  OutDataTypeStr=Inherit: Same as first input
  Product4 : Product  Inputs=4  SaturateOnIntegerOverflow=on  InputSameDT=on  OutDataTypeStr=Inherit: Same as first input
  RelHum2x : carnot/Basic/Material_Properties/RelHum2x
  Subsystem : Subsystem
  Sum : Sum  Inputs=-+  SaturateOnIntegerOverflow=on  InputSameDT=on  OutDataTypeStr=Inherit: Same as first input
  Sum1 : Sum  Inputs=-+  SaturateOnIntegerOverflow=on  InputSameDT=on  OutDataTypeStr=Inherit: Same as first input
  Sum2 : Sum  Inputs=++-  SaturateOnIntegerOverflow=on  InputSameDT=on  OutDataTypeStr=Inherit: Same as first input
  Terminator : Terminator
  cp Constant : Constant  Value=1006.8
  rho(CO2) / rho(air) * CO2norm (kg/kg) : Constant  Value=1.529*CO2norm
  "[S]" : Outport
  "[HVAC]" : Outport  Port=2
  wires:
  Fcn1/1 -> Sum2/1, Sum1/1
  Fcn/1 -> Sum1/2, Sum2/3
  Product2/1 -> Mux3/4  "mdot_H2O"
  Sum2/1 -> Product2/2  "x_sup"
  Product1/1 -> Sum2/2
  Sum1/1 -> Product1/2
  Constant5/1 -> Product1/1
  Subsystem/1(mdot_H2O) -> Terminator/1  "mdot_H2O"
  Constant4/1 -> Mux3/3
  Vdot/1 -> "1/h -> 1/s"/1
  Mux3/1 -> "[S]"/1
  Subsystem/2(mdot_CO2) -> Mux3/5  "mdot_CO2"
  WDB/1 -> Bus Selector/1
  AIB/1 -> Bus Selector1/1
  Density/1 -> Product3/2
  Bus Selector/3 -> RelHum2x/2, Density/2  "<Station_Pressure>"
  Bus Selector/2 -> RelHum2x/3  "<Relative_Humidity>"
  Bus Selector/1 -> RelHum2x/1, Density/1, Sum/2  "<Temperature_Ambient>"
  RelHum2x/1 -> Density/4, Mux4/1, Fcn1/1  "x_H2O"
  "\"air\""/1 -> Density/3
  Mux1/1 -> Subsystem/2(x_in)  "[x_H2O, x_CO2]_in"
  Bus Selector1/1 -> Sum/1  "<Tc>"
  Mux4/1 -> Subsystem/3(x_out)
  rho(CO2) / rho(air) * CO2norm (kg/kg)/1 -> Mux4/2  "x_CO2"
  Sum/1 -> Product4/2  "dT"
  cp Constant/1 -> Product4/3  "cp"
  Product3/1 -> Product4/4, Product2/1, Subsystem/1(mdot_air)
  Bus Selector1/2 -> Mux1/1, Fcn/1  "<x_H2O>"
  Bus Selector1/3 -> Mux1/2  "<x_CO2>"
  Constant/1 -> Mux3/2
  Constant1/1 -> Mux3/6
  Constant2/1 -> Mux3/8
  Constant3/1 -> Product4/1
  "1/h -> 1/s"/1 -> Product3/1
  Bus Creator1/1 -> "[HVAC]"/1
  Product4/1 -> Mux3/7, Integrator/1, Bus Creator1/1, Mux3/1  "ventilation power"
  Integrator/1 -> Bus Creator1/2  "ventilation energy"
